simulink model "sToPositionFcnBlock_th"  (R2018b)
settings: Solver=VariableStepAuto  StartTime=0.0  StopTime=1  RelTol=1e-3
values from neighbouring files (symbols this model uses):
  aB = 1    [courseFollow_plant_ts.m]    (also in plotdummy1.m)
  bB = 1    [courseFollow_plant_ts.m]    (also in plotdummy1.m)
  phi_curve = .5    (= 0.5)    [courseFollow_plant_ts.m]    (also in plotdummy1.m)
settings Model: Creator=James Reed  LastModifiedBy=James Reed

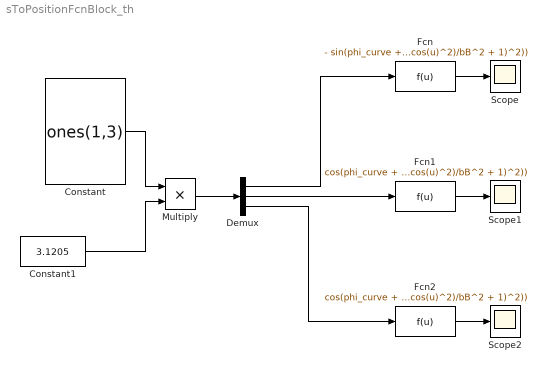
== system sToPositionFcnBlock_th ==
  Constant : Constant  Value=ones(1,3)
  Constant1 : Constant  Value=3.1205
  Demux : Demux  Outputs=3
  Fcn : Fcn  Expr=- sin(phi_curve + (aB^2*cos(u)*sin(u))/(bB^2*((aB^2*cos(u)^2)/bB^2 + 1)))*cos((aB*sin(u))/((aB^2*cos(u)^2)/bB^2 + 1))*((aB^2*cos(u)^2)/(bB^2*((aB^2*cos(u)^2)/bB^2 + 1)) - (aB^2*sin(u)^2)/(bB^2*((aB^2*cos(u)^2)/bB^2 + 1)) + (2*aB^4*cos(u)^2*sin(u)^2)/(bB^4*((aB^2*cos(u)^2)/bB^2 + 1)^2)) - cos(phi_curve + (aB^2*cos(u)*sin(u))/(bB^2*((aB^2*cos(u)^2)/bB^2 + 1)))*sin((aB*sin(u))/((aB^2*cos(u)^2)/bB^2 + 1))*((aB*cos(u))/((aB^2*cos(u)^2)/bB^2 + 1) + (2*aB^3*cos(u)*sin(u)^2)/(bB^2*((aB^2*cos(u)^2)/bB^2 + 1)^2))
  Fcn1 : Fcn  Expr=cos(phi_curve + (aB^2*cos(u)*sin(u))/(bB^2*((aB^2*cos(u)^2)/bB^2 + 1)))*cos((aB*sin(u))/((aB^2*cos(u)^2)/bB^2 + 1))*((aB*cos(u))/((aB^2*cos(u)^2)/bB^2 + 1) + (2*aB^3*cos(u)*sin(u)^2)/(bB^2*((aB^2*cos(u)^2)/bB^2 + 1)^2)) - sin(phi_curve + (aB^2*cos(u)*sin(u))/(bB^2*((aB^2*cos(u)^2)/bB^2 + 1)))*sin((aB*sin(u))/((aB^2*cos(u)^2)/bB^2 + 1))*((aB^2*cos(u)^2)/(bB^2*((aB^2*cos(u)^2)/bB^2 + 1)) - (aB^2*sin(u)^2)/(bB^2*((aB^2*cos(u)^2)/bB^2 + 1)) + (2*aB^4*cos(u)^2*sin(u)^2)/(bB^4*((aB^2*cos(u)^2)/bB^2 + 1)^2))
  Fcn2 : Fcn  Expr=cos(phi_curve + (aB^2*cos(u)*sin(u))/(bB^2*((aB^2*cos(u)^2)/bB^2 + 1)))*((aB^2*cos(u)^2)/(bB^2*((aB^2*cos(u)^2)/bB^2 + 1)) - (aB^2*sin(u)^2)/(bB^2*((aB^2*cos(u)^2)/bB^2 + 1)) + (2*aB^4*cos(u)^2*sin(u)^2)/(bB^4*((aB^2*cos(u)^2)/bB^2 + 1)^2))
  Multiply : Product
  Scope : Scope
  Scope1 : Scope
  Scope2 : Scope
  wires:
  Constant/1 -> Multiply/1
  Demux/3 -> Fcn2/1
  Demux/2 -> Fcn1/1
  Demux/1 -> Fcn/1
  Multiply/1 -> Demux/1
  Constant1/1 -> Multiply/2
  Fcn/1 -> Scope/1
  Fcn1/1 -> Scope1/1
  Fcn2/1 -> Scope2/1
